simulink model "receptorUSRP"  (R2025b)
settings: Solver=FixedStepDiscrete  StartTime=0.0  StopTime=7000  FixedStep=1/3312  RelTol=1e-3
libraries: commdigbbndpm3 x1, commfilt2 x1, commsdrhw_v2 x1, commcnvcod2 x1
settings Model: VariantFading=off  Creator=karolpalechor  LastModifiedBy=briyi

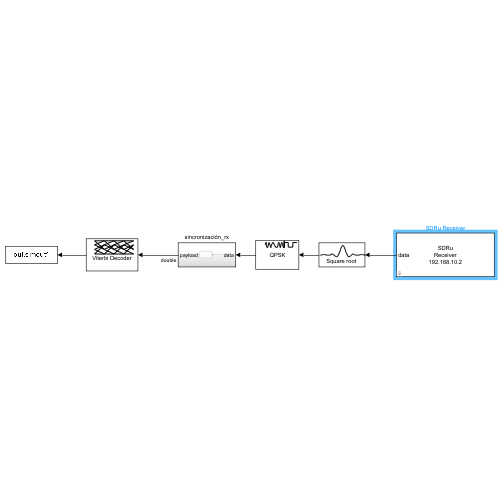
[thumbnail: Simulink's stored preview of the top-level diagram]
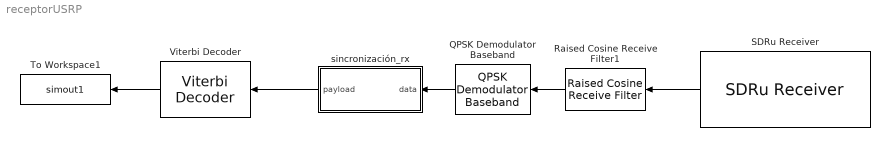
== system receptorUSRP ==
  QPSK Demodulator Baseband : commdigbbndpm3/QPSK Demodulator Baseband  OutType=Bit  DecType=Hard decision  VarSource=Dialog  Variance=1  Dec=Gray  Ph=pi/4  outDtype1=Inherit via internal rule  outDtype2=Inherit via internal rule  derotateFactorWordLen=16  derotateFactorDataTypeStr=Inherit: Same word length as input  derotateFactorLastDataTypeStr=Inherit: Same word length as input
  Raised Cosine Receive Filter1 : commfilt2/Raised Cosine Receive Filter  filtType=Square root  R=0.25  filtSpan=10  N=8  downFactor=8  downOffset=0  filterGain=1  InputProcessing=Columns as channels (frame based)  RateOptions=Enforce single-rate processing  framing=Mute  checkCoeff=off  variableName=rcRxFilt1  currentFiltSpan=10  D=5  inputOffset=0  sampMode=Mute  saveAsFlag=0  rateMode=Downsampling  checkGain=Normalized  launchFVT=on  roundingMode=Floor  overflowMode=off  coeffDataTypeStr=Inherit: Same word length as input  coeffMin=[]  coeffMax=[]  coeffLastDataTypeStr=Inherit: Same word length as input  accumDataTypeStr=Inherit: Same as product output  accumLastDataTypeStr=Inherit: Same as product output  outputDataTypeStr=Inherit: Same as accumulator  outputMin=[]  outputMax=[]  outputLastDataTypeStr=Inherit: Same as accumulator
  SDRu Receiver : commsdrhw_v2/SDRu Receiver  rxtx=rx  initializeIPAddress=0  devMap=10  USRP2_IP=192.168.10.2  USRP_IP_X300=192.168.10.2  USRP_IP_X310=192.168.10.2  USRP_IP_N300=192.168.10.2  USRP_IP_N310=192.168.10.2  USRP_IP_N320=192.168.10.2  USRP_IP_E320=192.168.10.2  USRP_IP_X410=192.168.10.2  USRP_serialNumB200=3136D21  USRP_serialNumB210=30F59A1  platform=N200/N210/USRP2  prevPlatform=N200/N210/USRP2  lastIPAddressPopup=192.168.10.2  USRP_ID=192.168.10.2  LastIPAddress=192.168.10.2  IsTwinRXDaughterboard=off  EnableTwinRXPhaseSync=off  losrc=0  ChannelMapping=1  rxAntennaPort=RX2  rxAntennaPortX410=RX1  centerFrequencySrc=Dialog  centerFrequency=2.45e9  loOffsetSrc=Dialog  loOffset=0  gainSrc=Dialog  gain=32  PPSSource=Internal  clockSource=Internal  EnableGPSLock=off  EnsureSyncGPSTime=off  EnableTimeTrigger=off  triggerTime=5  enableMIMOCableSync=off  EnableRefLock=off  masterClkRateParam=100e6  masterClkRateB200=32e6  masterClkRateB210=32e6  masterClkRateX300=200e6  masterClkRateX310=200e6  masterClkRateN300=125e6  masterClkRateN310=125e6  masterClkRateN320=200e6  masterClkRateE320=30.72e6  masterClkRateX410=250e6  masterClkRate=100e6  masterClkRateTwinRX=200e6  decimInterpSrc=Dialog  decimInterpPort=512  lastDecimSource=Dialog  decimInterp=512  USRP2_IP_NUM=[49 57 50 46 49 54 56 46 49 48 46 50]  sampleRate=195312.5  sampleTime=(512)/100000000  TransportDataType=int16  overrunUnderrunPort=off  dataLengthPort=off  EnableTimeStamps=off  outputDatatype=Same as transport data type  frameLength=362  HOST_DATA_PORT=0  HOST_CONTROL_PORT=0  USRP2_DATA_PORT=0  USRP2_CONTROL_PORT=0  bufferMode=Continuous streaming  EnableBurstMode=off  NumFramesInBurst=100
  To Workspace1 : ToWorkspace  VariableName=simout1  SaveFormat=Timeseries  SampleTime=-1
  Viterbi Decoder : commcnvcod2/Viterbi Decoder  trellis=poly2trellis(7,[171 133])  isPunctured=off  punctureVector=[1; 1; 0; 1; 0; 1]  erasures=off  dectype=Hard decision  nsdecb=3  runSigValErrCheck=off  tbdepth=34  opmode=Continuous  reset=off  delayedResetAction=off  smWordLength=16  outDataType=Inherit via internal rule
  sincronización_rx : Subsystem
  wires:
  sincronización_rx/1(payload) -> Viterbi Decoder/1
  Viterbi Decoder/1 -> To Workspace1/1
  QPSK Demodulator Baseband/1 -> sincronización_rx/1(data)
  Raised Cosine Receive Filter1/1 -> QPSK Demodulator Baseband/1
  SDRu Receiver/1 -> Raised Cosine Receive Filter1/1

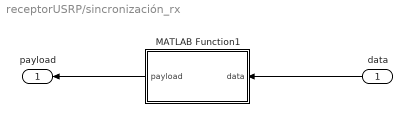
== system receptorUSRP/sincronización_rx ==
  data : Inport
  MATLAB Function1 : MATLAB Function  TreatAsAtomicUnit=on
  payload : Outport  OutDataTypeStr=double
  wires:
  MATLAB Function1/1(payload) -> payload/1
  data/1 -> MATLAB Function1/1(data)

== matlab function receptorUSRP/sincronización_rx/MATLAB Function1 ==
  data: data input; payload output
function payload = extract(data)
%#codegen
payload_len = int32(3312);
payload     = zeros(payload_len, 1, 'double');
sync_len    = int32(42);
data_len    = int32(length(data));

for j = int32(1):payload_len
    pos = sync_len + j;
    if pos <= data_len
        payload(j) = data(pos);
    end
end

end
